simulink model "inverseKinematics"  (R2017b)
settings: Solver=FixedStepDiscrete  StartTime=0.0  StopTime=tfsim  FixedStep=T  RelTol=1e-3  EnableMultiTasking=on
values from neighbouring files (symbols this model uses):
  Kp = diag([500 500 500 50])    [Approccio1.m]    (also in Approccio2.m = 10*diag([50 50 50 5]); Approccio3.m = 10*diag([50 50 50 5]); InversioneCinematica.m = diag([100 100 100 10]); PDpiuGravita.m = 1200*[1;1;1;1;1;1])
  q0 = [0 0 0 0 0 0]'    [Approccio1.m]    (also in Approccio2.m; Approccio3.m; main.m; main2.m)
  T = 0.001    [Approccio1.m]    (also in Approccio2.m; Approccio3.m; InversioneCinematica.m; MAIN_InitScript.m)
undefined symbols (not defined in the file or in its folder): cindirSchema, DiscIntNeverNeededParam, N, nullo, pinvJ
settings Model: Creator=Prova  LastModifiedBy=Prova
settings DataIOCC: LimitDataPoints=on
settings OptimizationCC: LifeSpan=inf
settings DebuggingCC: AllowSymbolicDim=off  SFUnexpectedBacktrackingDiag=warning  SFNoUnconditionalDefaultTransitionDiag=warning  SFExecutionAtInitializationDiag=none
settings ModelReferenceCC: PropagateSignalLabelsOutOfModel=off
settings CodeAppCC: StateflowObjectComments=on
settings GRTTargetCC: TargetLangStandard=C89/C90 (ANSI)
settings ConfigComp: CovMetricSettings=dw  CovHtmlReporting=on  CovSaveCumulativeToWorkspaceVar=on  CovSaveSingleToWorkspaceVar=on  CovExternalEMLEnable=off

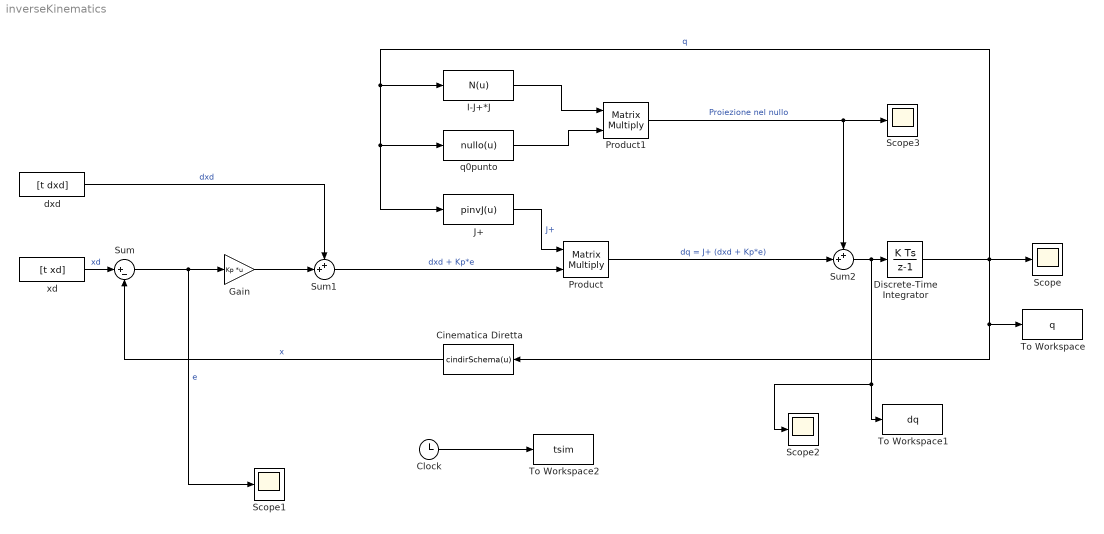
== system inverseKinematics ==
  Cinematica Diretta : MATLABFcn  MATLABFcn=cindirSchema(u)  OutputDimensions=[4,1]  Output1D=off
      mask Display: disp('K')
  Clock : Clock
  Discrete-Time Integrator : DiscreteIntegrator  InitialCondition=q0  InitialConditionSetting=State (most efficient)  SampleTime=T  ICPrevOutput=DiscIntNeverNeededParam  ICPrevScaledInput=DiscIntNeverNeededParam
  Gain : Gain  Gain=Kp  Multiplication=Matrix(K*u)
  I-J+*J : MATLABFcn  MATLABFcn=N(u)  OutputDimensions=[6,6]  Output1D=off
      mask Display: disp('N')
  J+ : MATLABFcn  MATLABFcn=pinvJ(u)  OutputDimensions=[6, 4]  Output1D=off
      mask Display: disp('J+')
  Product : Product  Multiplication=Matrix(*)
  Product1 : Product  Multiplication=Matrix(*)
  Scope{,1..3} (4 alike) : Scope
  Sum : Sum  Inputs=|+-
  Sum1 : Sum  Inputs=++|
  Sum2 : Sum  Inputs=++|
  To Workspace : ToWorkspace  VariableName=q  SampleTime=-1
  To Workspace1 : ToWorkspace  VariableName=dq  SampleTime=-1
  To Workspace2 : ToWorkspace  VariableName=tsim  SampleTime=-1
  dxd : FromWorkspace  VariableName=[t dxd]  SampleTime=0  OutputAfterFinalValue=Setting to zero
  "q0punto " : MATLABFcn  MATLABFcn=nullo(u)  OutputDimensions=[6,1]  Output1D=off
      mask Display: disp('q0')
  xd : FromWorkspace  VariableName=[t xd]  SampleTime=0  OutputAfterFinalValue=Holding final value
  wires:
  xd/1 -> Sum/1  "xd"
  Cinematica Diretta/1 -> Sum/2  "x"
  Sum/1 -> Scope1/1, Gain/1  "e"
  Gain/1 -> Sum1/2
  dxd/1 -> Sum1/1  "dxd"
  Sum1/1 -> Product/2  "dxd + Kp*e"
  J+/1 -> Product/1  "J+"
  Product/1 -> Sum2/2  "dq = J+ (dxd + Kp*e)"
  Clock/1 -> To Workspace2/1
  Discrete-Time Integrator/1 -> Scope/1, To Workspace/1, Cinematica Diretta/1, "q0punto "/1, J+/1, I-J+*J/1  "q"
  "q0punto "/1 -> Product1/2
  I-J+*J/1 -> Product1/1
  Sum2/1 -> Scope2/1, To Workspace1/1, Discrete-Time Integrator/1
  Product1/1 -> Sum2/1, Scope3/1  "Proiezione nel nullo"
